simulink model "teste2"  (R2012b)
settings: Solver=ode45  StartTime=0.0  StopTime=10  MaxStep=1e-4  RelTol=1e-3
undefined symbols (not defined in the file): default_fcem, Ke, L, R
libraries: Tools x4, simulink x4, BLDC x2
settings Model: Creator=h3now  LastModifiedBy=h3now

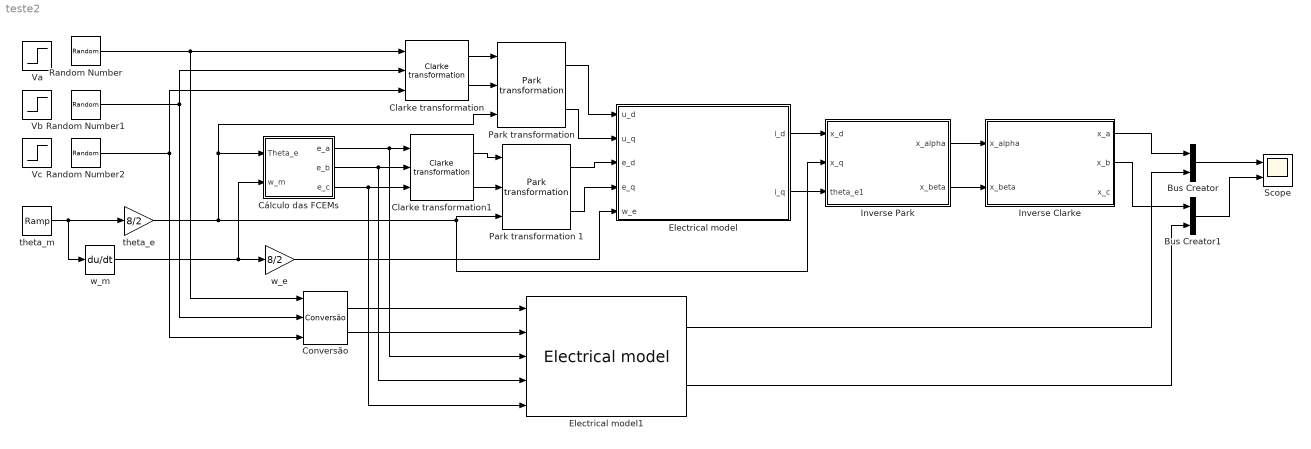
== system teste2 ==
  Bus Creator : BusCreator  Inputs=2
  Bus Creator1 : BusCreator  Inputs=2
  Clarke transformation : Tools/Clarke transformation
  Clarke transformation1 : Tools/Clarke transformation
  Conversão : BLDC/Conversão
  Cálculo das FCEMs : Subsystem
  Electrical model : Subsystem
  Electrical model1 : BLDC/BLDC/Electrical model
  Inverse Clarke : Subsystem
  Inverse Park : Subsystem
  "Park transformation " : Tools/Park transformation 
  Park transformation 1 : Tools/Park transformation 
  Random Number : RandomNumber  Variance=1000  SampleTime=1
  Random Number1 : RandomNumber  Variance=1000  Seed=1  SampleTime=1
  Random Number2 : RandomNumber  Variance=1000  Seed=2  SampleTime=1
  Scope : Scope  NumInputPorts=2
      settings: YMin=-5~-5  YMax=5~5
  Va : Step  Time=0  After=6  SampleTime=0
  Vb : Step  Time=0  After=6  SampleTime=0
  Vc : Step  Time=0  After=6  SampleTime=0
  theta_e : Gain  Gain=8/2
  theta_m : simulink/Sources/Ramp  slope=300  start=0  X0=0
  w_e : Gain  Gain=8/2
  w_m : Derivative
  wires:
  Conversão/1 -> Electrical model1/1
  Conversão/2 -> Electrical model1/2
  Cálculo das FCEMs/1(e_a) -> Electrical model1/3, Clarke transformation1/1
  Cálculo das FCEMs/2(e_b) -> Electrical model1/4, Clarke transformation1/2
  Cálculo das FCEMs/3(e_c) -> Electrical model1/5, Clarke transformation1/3
  Clarke transformation1/1 -> Park transformation 1/1
  Clarke transformation1/2 -> Park transformation 1/2
  Park transformation 1/1 -> Electrical model/3(e_d)
  Park transformation 1/2 -> Electrical model/4(e_q)
  "Park transformation "/1 -> Electrical model/1(u_d)
  "Park transformation "/2 -> Electrical model/2(u_q)
  Clarke transformation/1 -> "Park transformation "/1
  Clarke transformation/2 -> "Park transformation "/2
  Random Number/1 -> Conversão/1, Clarke transformation/1
  Random Number1/1 -> Clarke transformation/2, Conversão/2
  Random Number2/1 -> Clarke transformation/3, Conversão/3
  theta_m/1 -> theta_e/1, w_m/1
  w_m/1 -> w_e/1, Cálculo das FCEMs/2(w_m)
  w_e/1 -> Electrical model/5(w_e)
  theta_e/1 -> "Park transformation "/3, Cálculo das FCEMs/1(Theta_e), Park transformation 1/3, Inverse Park/3(theta_e1)
  Electrical model/1(i_d) -> Inverse Park/1(x_d)
  Electrical model/2(i_q) -> Inverse Park/2(x_q)
  Inverse Park/1("x_alpha ") -> Inverse Clarke/1(x_alpha)
  Inverse Park/2(x_beta) -> Inverse Clarke/2(x_beta)
  Inverse Clarke/1(x_a) -> Bus Creator/1
  Electrical model1/1 -> Bus Creator/2
  Bus Creator/1 -> Scope/1
  Inverse Clarke/2(x_b) -> Bus Creator1/1
  Electrical model1/2 -> Bus Creator1/2
  Bus Creator1/1 -> Scope/2

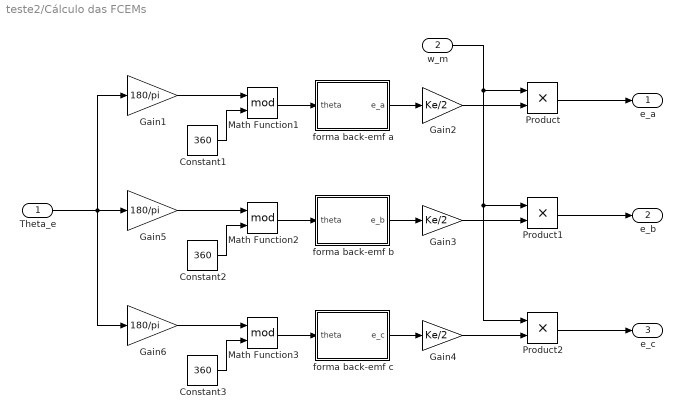
== system teste2/Cálculo das FCEMs ==
  Theta_e : Inport
  w_m : Inport  Port=2
  Constant1 : Constant  Value=360
  Constant2 : Constant  Value=360
  Constant3 : Constant  Value=360
  Gain1 : Gain  Gain=180/pi
  Gain2 : Gain  Gain=Ke/2
  Gain3 : Gain  Gain=Ke/2
  Gain4 : Gain  Gain=Ke/2
  Gain5 : Gain  Gain=180/pi
  Gain6 : Gain  Gain=180/pi
  Math Function1 : Math  Operator=mod  SaturateOnIntegerOverflow=on
  Math Function2 : Math  Operator=mod  SaturateOnIntegerOverflow=on
  Math Function3 : Math  Operator=mod  SaturateOnIntegerOverflow=on
  Product : Product  RndMeth=Zero
  Product1 : Product  RndMeth=Zero
  Product2 : Product  RndMeth=Zero
  forma back-emf a : Subsystem
  forma back-emf b : Subsystem
  forma back-emf c : Subsystem
  e_a : Outport
  e_b : Outport  Port=2
  e_c : Outport  Port=3
  wires:
  forma back-emf c/1(e_c) -> Gain4/1
  Math Function3/1 -> forma back-emf c/1(theta)
  forma back-emf b/1(e_b) -> Gain3/1
  Math Function2/1 -> forma back-emf b/1(theta)
  forma back-emf a/1(e_a) -> Gain2/1
  Math Function1/1 -> forma back-emf a/1(theta)
  Gain6/1 -> Math Function3/1
  Gain5/1 -> Math Function2/1
  Gain1/1 -> Math Function1/1
  Gain4/1 -> Product2/2
  Gain3/1 -> Product1/2
  w_m/1 -> Product2/1, Product1/1, Product/1
  Gain2/1 -> Product/2
  Product2/1 -> e_c/1
  Theta_e/1 -> Gain6/1, Gain1/1, Gain5/1
  Product1/1 -> e_b/1
  Product/1 -> e_a/1
  Constant1/1 -> Math Function1/2
  Constant2/1 -> Math Function2/2
  Constant3/1 -> Math Function3/2

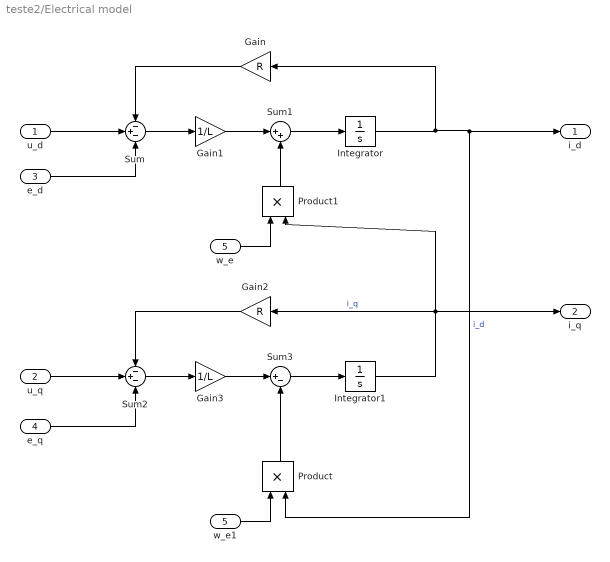
== system teste2/Electrical model ==
  u_d : Inport
  u_q : Inport  Port=2
  e_d : Inport  Port=3
  e_q : Inport  Port=4
  w_e : Inport  Port=5
  Gain : Gain  Gain=R
  Gain1 : Gain  Gain=1/L
  Gain2 : Gain  Gain=R
  Gain3 : Gain  Gain=1/L
  Integrator : Integrator
  Integrator1 : Integrator
  Product : Product  RndMeth=Zero
  Product1 : Product  RndMeth=Zero
  Sum : Sum  Inputs=-+-
  Sum1 : Sum  Inputs=|++
  Sum2 : Sum  Inputs=-+-
  Sum3 : Sum  Inputs=|+-
  w_e1 : InportShadow  Port=5
  i_d : Outport
  i_q : Outport  Port=2
  wires:
  Product/1 -> Sum3/2
  Sum3/1 -> Integrator1/1
  Gain3/1 -> Sum3/1
  Integrator1/1 -> i_q/1, Gain2/1, Product1/2  "i_q"
  Gain2/1 -> Sum2/1
  u_q/1 -> Sum2/2
  e_q/1 -> Sum2/3
  Sum2/1 -> Gain3/1
  Product1/1 -> Sum1/2
  Sum1/1 -> Integrator/1
  Integrator/1 -> i_d/1, Product/2, Gain/1  "i_d"
  e_d/1 -> Sum/3
  Gain/1 -> Sum/1
  Sum/1 -> Gain1/1
  Gain1/1 -> Sum1/1
  u_d/1 -> Sum/2
  w_e/1 -> Product1/1
  w_e1/1 -> Product/1

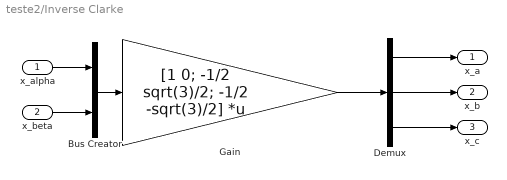
== system teste2/Inverse Clarke ==
  x_alpha : Inport
  x_beta : Inport  Port=2
  Bus Creator : BusCreator  Inputs=2
  Demux : Demux  Outputs=3
  Gain : Gain  Gain=[1 0; -1/2 sqrt(3)/2; -1/2 -sqrt(3)/2]  Multiplication=Matrix(K*u)
  x_a : Outport
  x_b : Outport  Port=2
  x_c : Outport  Port=3
  wires:
  Bus Creator/1 -> Gain/1
  Gain/1 -> Demux/1
  Demux/1 -> x_a/1
  Demux/2 -> x_b/1
  Demux/3 -> x_c/1
  x_beta/1 -> Bus Creator/2
  x_alpha/1 -> Bus Creator/1

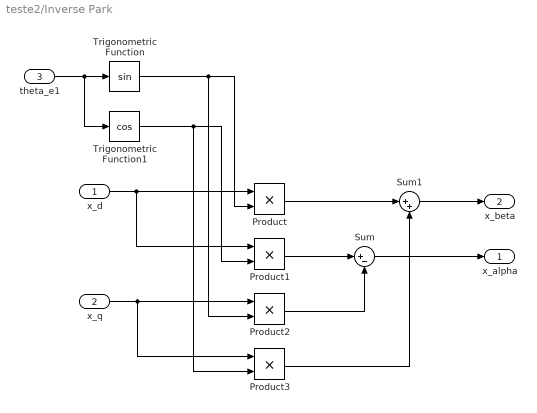
== system teste2/Inverse Park ==
  x_d : Inport
  x_q : Inport  Port=2
  theta_e1 : Inport  Port=3
  Product{,1..3} (4 alike) : Product  RndMeth=Zero
  Sum : Sum  Inputs=|+-
  Sum1 : Sum  Inputs=|++
  Trigonometric Function : Trigonometry  OutputSignalType=real
  Trigonometric Function1 : Trigonometry  Operator=cos  OutputSignalType=real
  "x_alpha " : Outport
  x_beta : Outport  Port=2
  wires:
  Product/1 -> Sum1/1
  Sum1/1 -> x_beta/1
  theta_e1/1 -> Trigonometric Function1/1, Trigonometric Function/1
  x_d/1 -> Product/1, Product1/1
  Sum/1 -> "x_alpha "/1
  Trigonometric Function/1 -> Product2/2, Product/2
  Product3/1 -> Sum1/2
  Product2/1 -> Sum/2
  Trigonometric Function1/1 -> Product3/2, Product1/2
  x_q/1 -> Product3/1, Product2/1
  Product1/1 -> Sum/1

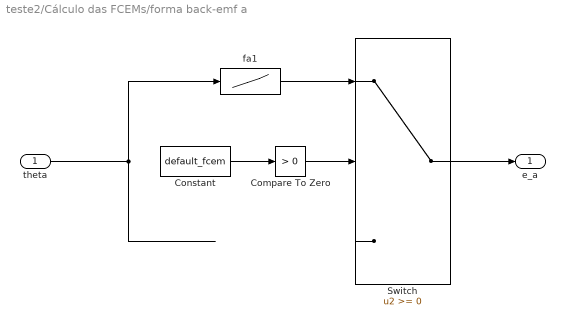
== system teste2/Cálculo das FCEMs/forma back-emf a ==
  theta : Inport
  Compare To Zero : simulink/Logic and Bit Operations/Compare To Zero  relop=>  OutDataTypeStr=boolean
  Constant : Constant  Value=default_fcem
  Switch : Switch
  fa1 : Lookup  InputValues=[0 30 60 90 120 150 180 210 240 270 300 330 360]  Table=[ 1 1 1 0 -1 -1 -1 -1 -1 0 1 1 1]
  e_a : Outport
  wires:
  Constant/1 -> Compare To Zero/1
  Compare To Zero/1 -> Switch/2
  ? -> Switch/3
  fa1/1 -> Switch/1
  Switch/1 -> e_a/1
  theta/1 -> fa1/1

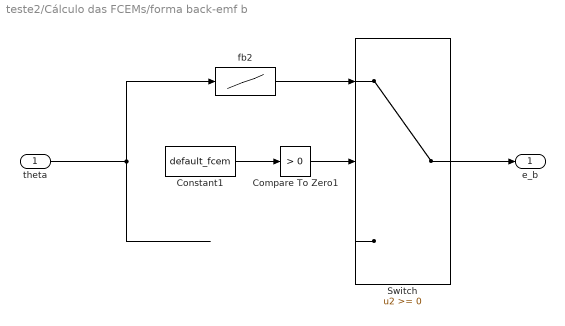
== system teste2/Cálculo das FCEMs/forma back-emf b ==
  theta : Inport
  Compare To Zero1 : simulink/Logic and Bit Operations/Compare To Zero  relop=>  OutDataTypeStr=boolean
  Constant1 : Constant  Value=default_fcem
  Switch : Switch
  fb2 : Lookup  InputValues=[0 30 60 90 120 150 180 210 240 270 300 330 360]  Table=[-1 0 1 1 1 1 1 0 -1 -1 -1 -1 -1]
  e_b : Outport
  wires:
  fb2/1 -> Switch/1
  Switch/1 -> e_b/1
  Constant1/1 -> Compare To Zero1/1
  Compare To Zero1/1 -> Switch/2
  theta/1 -> fb2/1
  ? -> Switch/3

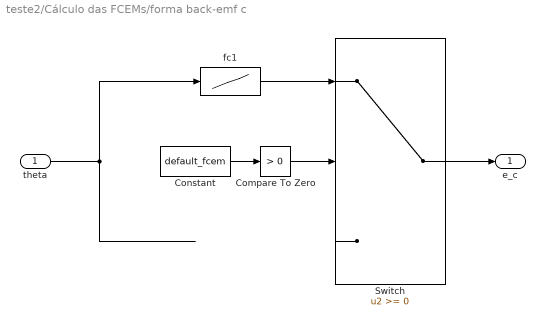
== system teste2/Cálculo das FCEMs/forma back-emf c ==
  theta : Inport
  Compare To Zero : simulink/Logic and Bit Operations/Compare To Zero  relop=>  OutDataTypeStr=boolean
  Constant : Constant  Value=default_fcem
  Switch : Switch
  fc1 : Lookup  InputValues=[0 30 60 90 120 150 180 210 240 270 300 330 360]  Table=[-1 -1 -1 -1 -1 0 1 1 1 1 1 0 -1]
  e_c : Outport
  wires:
  fc1/1 -> Switch/1
  Switch/1 -> e_c/1
  Constant/1 -> Compare To Zero/1
  Compare To Zero/1 -> Switch/2
  theta/1 -> fc1/1
  ? -> Switch/3
